simulink library "calcPathCoords"  (R2020a)
settings: Solver=VariableStepAuto  StartTime=0.0  StopTime=10.0  RelTol=1e-3
settings Model: Creator=Ayaz  LastModifiedBy=Ayaz

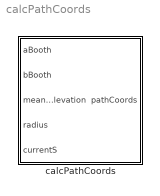
== system calcPathCoords ==
  calcPathCoords : Subsystem

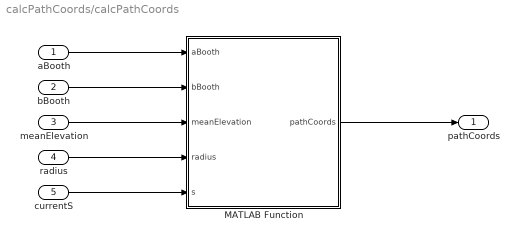
== system calcPathCoords/calcPathCoords ==
  aBooth : Inport
  bBooth : Inport  Port=2
  meanElevation : Inport  Port=3
  radius : Inport  Port=4
  currentS : Inport  Port=5
  MATLAB Function : MATLAB Function  TreatAsAtomicUnit=on
  pathCoords : Outport
  wires:
  MATLAB Function/1(pathCoords) -> pathCoords/1
  meanElevation/1 -> MATLAB Function/3(meanElevation)
  bBooth/1 -> MATLAB Function/2(bBooth)
  radius/1 -> MATLAB Function/4(radius)
  aBooth/1 -> MATLAB Function/1(aBooth)
  currentS/1 -> MATLAB Function/5(s)

== matlab function calcPathCoords/MATLAB Function ==
  data: aBooth input; pathCoords output; bBooth input; meanElevation input; radius input; s input
function pathCoords = getPathCoords(aBooth,bBooth,meanElevation,radius,s)

pathCoords = getPathCoords(aBooth,bBooth,meanElevation,radius,s);

end
